simulink model "VirtualModel_04_2019"  (Simulink 9.3)
settings: Solver=VariableStepAuto  StartTime=0.0  StopTime=10.0  RelTol=1e-3
values from neighbouring files (symbols this model uses):
  A = (m_t/2+m_tr+m_ts)*l_t    (= 0.0946875)    [Final_val.m]
  B = (m_m/2+m_mr+m_ms)*l_m    (= 0.11046)    [Final_val.m]
  C = (m_b/2*l_b+m_cb*l_cb)    (= 0.02054)    [Final_val.m]
  D = (m_b/3*l_b^2+m_cb*l_cb^2)    (= 0.00509253333333)    [Final_val.m]
  E = (m_m/3+m_mr+m_ms)*l_m^2+(m_t/3+m_tr+m_ts)*l_t^2    (= 0.0498816166667)    [Final_val.m]
  F = m_ms*r_ms^2+m_ts/2*r_ts^2    (= 0.006230625)    [Final_val.m]
  g = 9.81    [Final_val.m]
  J_mr = 2.65e-5    (= 2.65e-05)    [Final_val.m]
  J_tr = 1.654e-5    (= 1.654e-05)    [Final_val.m]
  J_v = Jv1+Jv2+Jv3+Jv4+Jv5+Jv6+Jv7+Jv8    (= 0.0593269625)    [Final_val.m]
  k_h = 0.0095    [Final_val.m]
  k_v = 0.00545    [Final_val.m]
  l_b = 0.26    [Final_val.m]
  l_m = 0.24    [Final_val.m]
  l_t = 0.25    [Final_val.m]
  polynom =     [polynom.mat]
  Tm = 0.8921    [Final_val.m]
  Tt = 0.3423    [Final_val.m]
libraries: simulink_extras x2, vrlib x1
settings Model: Creator=e0371305  LastModifiedBy=Joy
settings DataIOCC: SaveFormat=Dataset  SignalLoggingSaveFormat=Dataset
settings OptimizationCC: LifeSpan=auto
settings DebuggingCC: UnderspecifiedInitializationDetection=Simplified  MergeDetectMultiDrivingBlocksExec=error  FcnCallInpInsideContextMsg=error  SFUnexpectedBacktrackingDiag=error  SFNoUnconditionalDefaultTransitionDiag=error  SFExecutionAtInitializationDiag=warning
settings HardwareCC: ProdBitPerPointer=64  ProdBitPerSizeT=64  ProdBitPerPtrDiffT=64  ProdLargestAtomicFloat=Float  ProdIntDivRoundTo=Zero  ProdEndianess=LittleEndian  ProdWordSize=64  ProdHWDeviceType=Intel->x86-64 (Windows64)
settings ModelReferenceCC: PropagateSignalLabelsOutOfModel=on
settings GRTTargetCC: TargetLangStandard=C99 (ISO)  CombineOutputUpdateFcns=on  GRTInterface=off
settings ConfigComp: CovMetricSettings=dwe  CovSaveCumulativeToWorkspaceVar=off  CovSaveSingleToWorkspaceVar=off  CovExternalEMLEnable=on

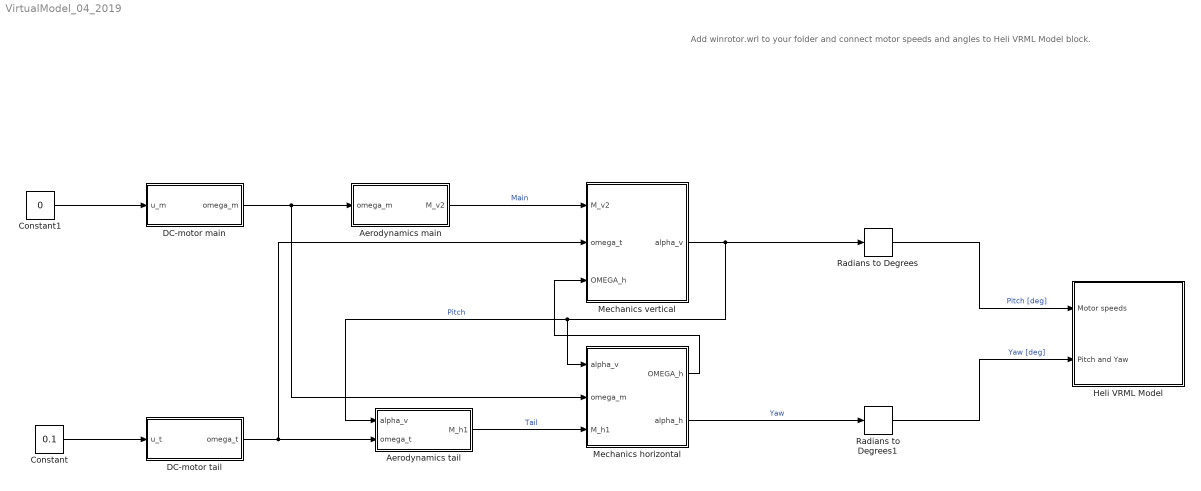
== system VirtualModel_04_2019 ==
  note: Add winrotor.wrl to your folder
      | and connect motor speeds and angles to Heli VRML Model block.
  Aerodynamics main : Subsystem
  Aerodynamics tail : Subsystem
  Constant : Constant  Value=0.1
  Constant1 : Constant  Value=0  VectorParams1D=off
  DC-motor main : Subsystem
  DC-motor tail : Subsystem
  Heli VRML Model : Subsystem
  Mechanics horizontal : Subsystem
  Mechanics vertical : Subsystem
  Radians to Degrees : simulink_extras/Transformations/Radians to Degrees
  Radians to Degrees1 : simulink_extras/Transformations/Radians to Degrees
  wires:
  DC-motor tail/1(omega_t) -> Aerodynamics tail/2(omega_t), Mechanics vertical/2(omega_t)
  DC-motor main/1(omega_m) -> Aerodynamics main/1(omega_m), Mechanics horizontal/2(omega_m)
  Mechanics horizontal/1(OMEGA_h) -> Mechanics vertical/3(OMEGA_h)
  Mechanics vertical/1(alpha_v) -> Radians to Degrees/1, Aerodynamics tail/1(alpha_v), Mechanics horizontal/1(alpha_v)  "Pitch"
  Mechanics horizontal/2(alpha_h) -> Radians to Degrees1/1  "Yaw"
  Aerodynamics main/1(M_v2) -> Mechanics vertical/1(M_v2)  "Main"
  Radians to Degrees/1 -> Heli VRML Model/1(Motor speeds)  "Pitch [deg]"
  Aerodynamics tail/1(M_h1) -> Mechanics horizontal/3(M_h1)  "Tail"
  Radians to Degrees1/1 -> Heli VRML Model/2(Pitch and Yaw)  "Yaw [deg]"
  Constant1/1 -> DC-motor main/1(u_m)
  Constant/1 -> DC-motor tail/1(u_t)

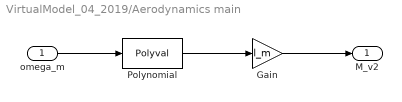
== system VirtualModel_04_2019/Aerodynamics main ==
  omega_m : Inport
  Gain : Gain  Gain=l_m
  Polynomial : Polyval  Coefs=polynom.MainForce
  M_v2 : Outport  VectorParamsAs1DForOutWhenUnconnected=off
  wires:
  omega_m/1 -> Polynomial/1
  Gain/1 -> M_v2/1
  Polynomial/1 -> Gain/1

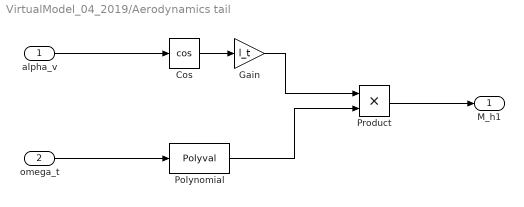
== system VirtualModel_04_2019/Aerodynamics tail ==
  alpha_v : Inport
  omega_t : Inport  Port=2
  Cos : Trigonometry  Operator=cos
  Gain : Gain  Gain=l_t
  Polynomial : Polyval  Coefs=polynom.TailForce
  Product : Product
  M_h1 : Outport  VectorParamsAs1DForOutWhenUnconnected=off
  wires:
  Product/1 -> M_h1/1
  Gain/1 -> Product/1
  Polynomial/1 -> Product/2
  Cos/1 -> Gain/1
  alpha_v/1 -> Cos/1
  omega_t/1 -> Polynomial/1

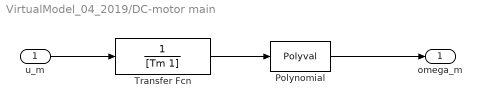
== system VirtualModel_04_2019/DC-motor main ==
  u_m : Inport
  Polynomial : Polyval  Coefs=polynom.MainSpeed
  Transfer Fcn : TransferFcn  Denominator=[Tm 1]
  omega_m : Outport  VectorParamsAs1DForOutWhenUnconnected=off
  wires:
  u_m/1 -> Transfer Fcn/1
  Polynomial/1 -> omega_m/1
  Transfer Fcn/1 -> Polynomial/1

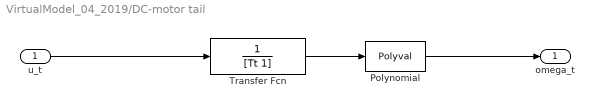
== system VirtualModel_04_2019/DC-motor tail ==
  u_t : Inport
  Polynomial : Polyval  Coefs=polynom.TailSpeed
  Transfer Fcn : TransferFcn  Denominator=[Tt 1]
  omega_t : Outport  VectorParamsAs1DForOutWhenUnconnected=off
  wires:
  u_t/1 -> Transfer Fcn/1
  Polynomial/1 -> omega_t/1
  Transfer Fcn/1 -> Polynomial/1

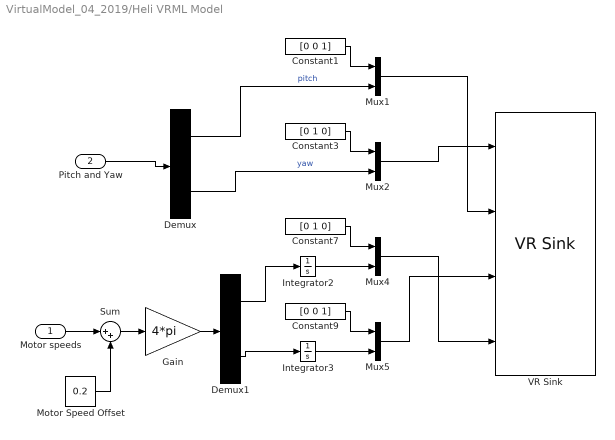
== system VirtualModel_04_2019/Heli VRML Model ==
  Motor speeds : Inport
  Pitch and Yaw : Inport  Port=2
  Constant1 : Constant  Value=[0 0 1]
  Constant3 : Constant  Value=[0 1 0]
  Constant7 : Constant  Value=[0 1 0]
  Constant9 : Constant  Value=[0 0 1]
  Demux : Demux  Outputs=2
  Demux1 : Demux  Outputs=2
  Gain : Gain  Gain=4*pi
  Integrator2 : Integrator
  Integrator3 : Integrator
  Motor Speed Offset : Constant  Value=0.2
  Mux{1..2,4..5} (4 alike) : Mux  Inputs=2
  Sum : Sum  Inputs=|++
  VR Sink : vrlib/VR Sink  InstantiateOnLoad=on  SampleTime=0.1  ViewEnable=on  RemoteChange=off  RemoteView=off  FieldsWritten=YAW.rotation.4.1.1.double#PITCH.rotation.4.1.1.double#TAILPROP.rotation.4.1.1.double#MAINPROP.rotation.4.1.1.double  WorldFileName=twinrotor.wrl  AutoView=on  VideoDimensions=[]  AllowVariableSize=off  FigureProperties="{'Position', 'Name', 'Viewpoint', 'CameraBound', 'CameraDirection', 'CameraPosition', 'CameraUpVector', 'ZoomFactor', 'Antialiasing', 'Headlight', 'Lighting', 'NavPanel', 'Sound', 'StatusBar', 'Stereo3D', 'Stereo3DCameraOffset', 'Stereo3DHIT', 'ToolBar', 'Textures', 'Transparency', 'Triad', 'Wireframe', 'NavZones', 'NavMode', 'NavSpeed', 'CaptureFileFormat', 'CaptureFileName', 'Record2DCompressMethod', 'Record2DCompressQuality', 'Record2D', 'Record2DFileName', 'Record2DFPS'; [5.0000000000000000e+00   9.2000000000000000e+01   5.7600000000000000e+02   3.5000000000000000e+02], '', 'View1', 'on', [0.0000000000000000e+00   0.0000000000000000e+00  -1.0000000000000000e+00], [0.0000000000000000e+00   0.0000000000000000e+00   0.0000000000000000e+00], [0.0000000000000000e+00   1.0000000000000000e+00   0.0000000000000000e+00], [1.0000000000000000e+00], 'on', 'off', 'on', 'halfbar', 'on', 'on', 'off', [1.0000000149011612e-01], [0.0000000000000000e+00], 'on', 'on', 'on', 'none', 'off', 'off', 'walk', 'normal', 'tif', '%f_anim_%n.tif', 'auto', [7.5000000000000000e+01], 'off', '%f_anim_%n.avi', 'auto'}"
  wires:
  Constant1/1 -> Mux1/1
  Constant3/1 -> Mux2/1
  Constant7/1 -> Mux4/1
  Constant9/1 -> Mux5/1
  Integrator2/1 -> Mux4/2
  Integrator3/1 -> Mux5/2
  Demux/1 -> Mux1/2  "pitch"
  Demux1/1 -> Integrator2/1
  Demux1/2 -> Integrator3/1
  Pitch and Yaw/1 -> Demux/1
  Demux/2 -> Mux2/2  "yaw"
  Gain/1 -> Demux1/1
  Sum/1 -> Gain/1
  Motor speeds/1 -> Sum/1
  Motor Speed Offset/1 -> Sum/2
  Mux4/1 -> VR Sink/4
  Mux5/1 -> VR Sink/3
  Mux2/1 -> VR Sink/1
  Mux1/1 -> VR Sink/2

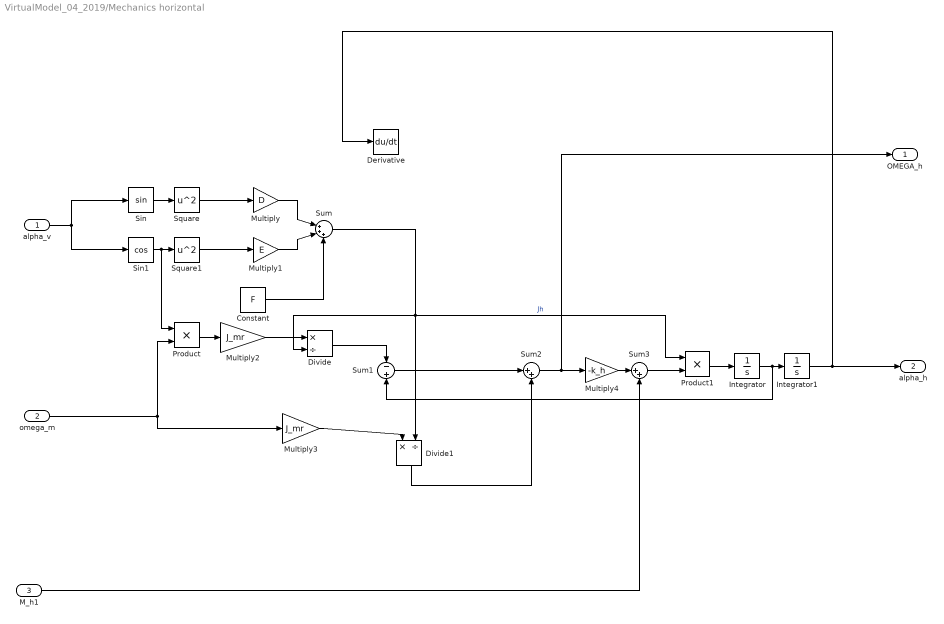
== system VirtualModel_04_2019/Mechanics horizontal ==
  alpha_v : Inport
  omega_m : Inport  Port=2
  M_h1 : Inport  Port=3
  Constant : Constant  Value=F
  Derivative : Derivative
  Divide : Product  Inputs=*/
  Divide1 : Product  Inputs=*/
  Integrator : Integrator
  Integrator1 : Integrator
  Multiply : Gain  Gain=D
  Multiply1 : Gain  Gain=E
  Multiply2 : Gain  Gain=J_mr
  Multiply3 : Gain  Gain=J_mr
  Multiply4 : Gain  Gain=-k_h
  Product : Product
  Product1 : Product
  Sin : Trigonometry
  Sin1 : Trigonometry  Operator=cos
  Square : Math  Operator=square  SaturateOnIntegerOverflow=on
  Square1 : Math  Operator=square  SaturateOnIntegerOverflow=on
  Sum : Sum  Inputs=|+++
  Sum1 : Sum  Inputs=-+
  Sum2 : Sum  Inputs=|++
  Sum3 : Sum  Inputs=|++
  OMEGA_h : Outport  VectorParamsAs1DForOutWhenUnconnected=off
  alpha_h : Outport  Port=2  VectorParamsAs1DForOutWhenUnconnected=off
  wires:
  Divide/1 -> Sum1/1
  Integrator1/1 -> alpha_h/1, Derivative/1
  Integrator/1 -> Integrator1/1, Sum1/2
  Product1/1 -> Integrator/1
  Sum3/1 -> Product1/2
  M_h1/1 -> Sum3/2
  Multiply4/1 -> Sum3/1
  Sum2/1 -> Multiply4/1, OMEGA_h/1
  Divide1/1 -> Sum2/2
  Sum1/1 -> Sum2/1
  Multiply3/1 -> Divide1/1
  Sum/1 -> Divide/2, Divide1/2, Product1/1  "Jh"
  Multiply2/1 -> Divide/1
  Product/1 -> Multiply2/1
  omega_m/1 -> Multiply3/1, Product/2
  Constant/1 -> Sum/3
  Multiply1/1 -> Sum/2
  Multiply/1 -> Sum/1
  Square/1 -> Multiply/1
  Square1/1 -> Multiply1/1
  Sin/1 -> Square/1
  Sin1/1 -> Square1/1, Product/1
  alpha_v/1 -> Sin1/1, Sin/1

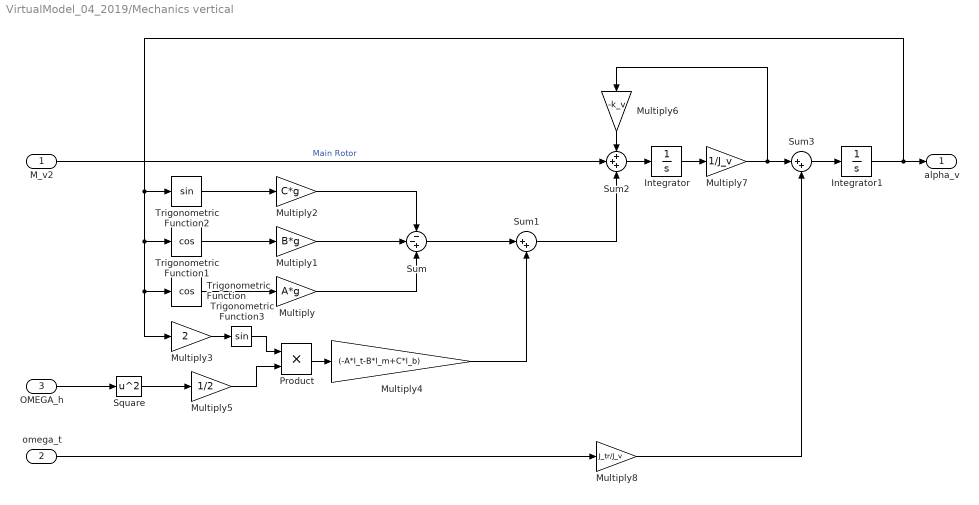
== system VirtualModel_04_2019/Mechanics vertical ==
  M_v2 : Inport
  omega_t : Inport  Port=2
  OMEGA_h : Inport  Port=3
  Integrator : Integrator
  Integrator1 : Integrator
  Multiply : Gain  Gain=A*g
  Multiply1 : Gain  Gain=B*g
  Multiply2 : Gain  Gain=C*g
  Multiply3 : Gain  Gain=2
  Multiply4 : Gain  Gain=(-A*l_t-B*l_m+C*l_b)
  Multiply5 : Gain  Gain=1/2
  Multiply6 : Gain  Gain=-k_v
  Multiply7 : Gain  Gain=1/J_v
  Multiply8 : Gain  Gain=J_tr/J_v
  Product : Product
  Square : Math  Operator=square  SaturateOnIntegerOverflow=on
  Sum : Sum  Inputs=--+
  Sum1 : Sum  Inputs=|++
  Sum2 : Sum  Inputs=+++
  Sum3 : Sum  Inputs=|++
  Trigonometric Function : Trigonometry  Operator=cos
  Trigonometric Function1 : Trigonometry  Operator=cos
  Trigonometric Function2 : Trigonometry
  Trigonometric Function3 : Trigonometry
  alpha_v : Outport  VectorParamsAs1DForOutWhenUnconnected=off
  wires:
  Integrator1/1 -> alpha_v/1, Multiply3/1, Trigonometric Function/1, Trigonometric Function1/1, Trigonometric Function2/1
  Sum3/1 -> Integrator1/1
  Product/1 -> Multiply4/1
  Trigonometric Function3/1 -> Product/1
  Multiply5/1 -> Product/2
  Multiply8/1 -> Sum3/2
  Multiply7/1 -> Multiply6/1, Sum3/1
  Sum2/1 -> Integrator/1
  Integrator/1 -> Multiply7/1
  Multiply6/1 -> Sum2/1
  M_v2/1 -> Sum2/2  "Main Rotor"
  Sum1/1 -> Sum2/3
  Sum/1 -> Sum1/1
  Multiply4/1 -> Sum1/2
  Square/1 -> Multiply5/1
  OMEGA_h/1 -> Square/1
  Multiply3/1 -> Trigonometric Function3/1
  Multiply/1 -> Sum/3
  Multiply1/1 -> Sum/2
  Multiply2/1 -> Sum/1
  Trigonometric Function2/1 -> Multiply2/1
  Trigonometric Function1/1 -> Multiply1/1
  Trigonometric Function/1 -> Multiply/1
  omega_t/1 -> Multiply8/1
